simulink model "transformerlesspv0002"  (Simulink 9.2)
settings: Solver=ode45  StartTime=0.0  StopTime=2  RelTol=1e-3  EnableMultiTasking=on
undefined symbols (not defined in the file): dEgdT, EgRef, gcbh, k1, Rsh_array5pc, sps_rtmsupport, Tref_K, Ts_Control, VT_ref
libraries: powerlib x40, spsPVarrayModel x3, simulink x1, simulink_extras x1
(part 6 of 6)

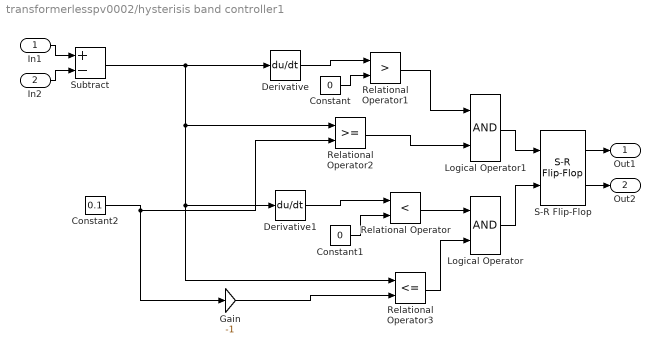
== system transformerlesspv0002/hysterisis band controller1 ==
  In1 : Inport
  In2 : Inport  Port=2
  Constant : Constant  Value=0
  Constant1 : Constant  Value=0
  Constant2 : Constant  Value=0.1
  Derivative : Derivative
  Derivative1 : Derivative
  Gain : Gain  Gain=-1
  Logical Operator : Logic  AllPortsSameDT=off  OutDataTypeStr=boolean
  Logical Operator1 : Logic  AllPortsSameDT=off  OutDataTypeStr=boolean
  Relational Operator : RelationalOperator  Operator=<  OutDataTypeStr=boolean  RndMeth=Nearest
  Relational Operator1 : RelationalOperator  Operator=>  OutDataTypeStr=boolean  RndMeth=Nearest
  Relational Operator2 : RelationalOperator  OutDataTypeStr=boolean  RndMeth=Nearest
  Relational Operator3 : RelationalOperator  Operator=<=  OutDataTypeStr=boolean  RndMeth=Nearest
  S-R Flip-Flop : simulink_extras/Flip Flops/S-R Flip-Flop  initial_condition=1
  Subtract : Sum  Inputs=+-
  Out1 : Outport
  Out2 : Outport  Port=2
  wires:
  Derivative/1 -> Relational Operator1/1
  Constant/1 -> Relational Operator1/2
  Derivative1/1 -> Relational Operator/1
  Constant1/1 -> Relational Operator/2
  Subtract/1 -> Derivative1/1, Relational Operator3/1, Relational Operator2/1, Derivative/1
  Relational Operator1/1 -> Logical Operator1/1
  Relational Operator2/1 -> Logical Operator1/2
  Relational Operator/1 -> Logical Operator/1
  Relational Operator3/1 -> Logical Operator/2
  Gain/1 -> Relational Operator3/2
  Constant2/1 -> Relational Operator2/2, Gain/1
  Logical Operator1/1 -> S-R Flip-Flop/1
  Logical Operator/1 -> S-R Flip-Flop/2
  In1/1 -> Subtract/1
  S-R Flip-Flop/1 -> Out1/1
  In2/1 -> Subtract/2
  S-R Flip-Flop/2 -> Out2/1

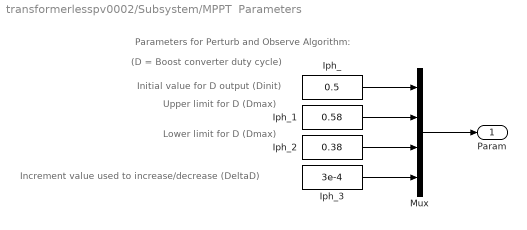
== system transformerlesspv0002/Subsystem/MPPT  Parameters ==
  note: Upper limit for D (Dmax)
  note: Increment value used to increase/decrease (DeltaD)
  note: Initial value for D output (Dinit)
  note: (D = Boost converter duty cycle)
  note: Lower limit for D (Dmax)
  note: Parameters for Perturb and Observe Algorithm:
  Iph_ : Constant  Value=0.5
  Iph_1 : Constant  Value=0.58
  Iph_2 : Constant  Value=0.38
  Iph_3 : Constant  Value=3e-4
  Mux : Mux
  Param : Outport
  wires:
  Iph_/1 -> Mux/1
  Iph_1/1 -> Mux/2
  Iph_2/1 -> Mux/3
  Iph_3/1 -> Mux/4
  Mux/1 -> Param/1

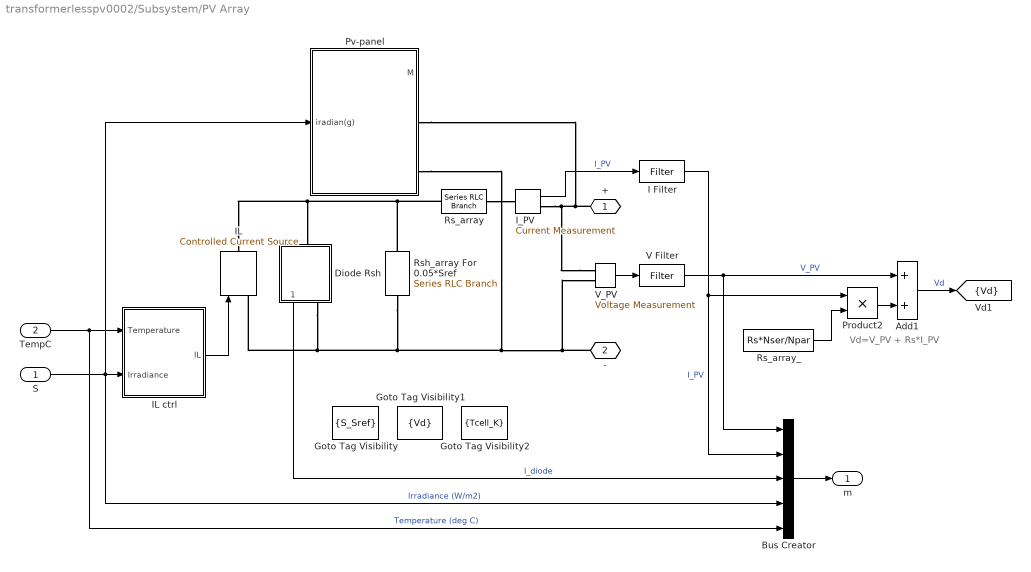
== system transformerlesspv0002/Subsystem/PV Array ==
  note: Vd=V_PV + Rs*I_PV
  S : Inport
  TempC : Inport  Port=2
  Add1 : Sum
  Bus Creator : BusCreator  Inputs=5
  Diode Rsh : Subsystem
      mask Display:
      | plot(-75,-50,100,150, [-15 -15 43 -15 -15 -75],[50 8 50 92 50 50], ...
      |     [43 43],[8 94],[100 43], [50 50])
  Goto Tag Visibility : GotoTagVisibility  GotoTag=S_Sref
  Goto Tag Visibility1 : GotoTagVisibility  GotoTag=Vd
  Goto Tag Visibility2 : GotoTagVisibility  GotoTag=Tcell_K
  I Filter : spsPVarrayModel/Filter  SystemSampleTime=-1  VariantControl=Variant1
  IL : powerlib/Electrical Sources/Controlled Current Source  Initialize=on  Source_Type=AC  Amplitude=0  Phase=0  Frequency=0  Measurements=None
      settings: SourceProductName=Simscape Electrical
  IL ctrl : Subsystem
  I_PV : powerlib/Measurements/Current Measurement  PhasorSimulation=off  OutputType=Complex  PSBequivalent=0
      settings: SourceProductName=Simscape Electrical
  Product2 : Product  Inputs=**  RndMeth=Zero
  Pv-panel : Subsystem  mask(PV_PANEL){Ns=600, Np=66}
      mask prompts: Ns "Number_of_series_connectd_pvcells"; Np "Number_of_parallel_connected_strings"
      mask help: THIS BLOCK IMPLEMENTS PHOTO VOLTAIC PANEL.NUMBER OF SERIES PV CELLS CAN BE CONTROLLED AND NUMBER OF PARALLEL STRINGS 0F PV CELLS CAN BE CONTROLLED
      mask init:
      | u=1.5;%diode 
      | k=1.3806e-23;%boltzman constant
      | T=298;%room temp
      | q=1.6022e-19;%charge
      | vt=(u*k*T)/q;
      | Vt_panel=vt*Ns;
      | Iph=8;
      | Iph_panel=Iph*Np;
      | I0=9.845e-7;
      | I0_panel=I0*Np;
      | Rs=0.001;
      | Rs_panel=Rs*(Ns/Np);
      | Rsh=142.94;
      | Rsh_panel=Rsh*(Ns/Np);
      | G0=1000;
      mask Display: image(imread('pv_panel.jpg'))
  Rs_array : powerlib/Elements/Series RLC Branch  LConnTagsString=__new0  RConnTagsString=__new0  BranchType=R  Resistance=Rs*Nser/Npar  Inductance=1e-3  SetiL0=off  InitialCurrent=0  Capacitance=1e-6  Setx0=off  InitialVoltage=0  Measurements=None
      settings: SourceProductName=Simscape Electrical
  Rs_array_ : Constant  Value=Rs*Nser/Npar
  Rsh_array For 0.05*Sref : powerlib/Elements/Series RLC Branch  LConnTagsString=__new0  RConnTagsString=__new0  BranchType=R  Resistance=Rsh_array5pc  Inductance=1e-3  SetiL0=off  InitialCurrent=0  Capacitance=1e-6  Setx0=off  InitialVoltage=0  Measurements=None
      settings: SourceProductName=Simscape Electrical
  V Filter : spsPVarrayModel/Filter  SystemSampleTime=-1  VariantControl=Variant1
  V_PV : powerlib/Measurements/Voltage Measurement  PhasorSimulation=off  OutputType=Complex  PSBequivalent=0
      settings: SourceProductName=Simscape Electrical
  + : PMIOPort  Side=Right
  - : PMIOPort  Port=2  Side=Right
  m : Outport
  tag scope: Vd=scoped
  wires:
  V Filter/1 -> Add1/1, Bus Creator/1  "V_PV"
  I Filter/1 -> Product2/1, Bus Creator/2  "I_PV"
  V_PV/1 -> V Filter/1
  IL ctrl/1(IL) -> IL/1
  Bus Creator/1 -> m/1
  Rs_array_/1 -> Product2/2
  Product2/1 -> Add1/2
  I_PV/1 -> I Filter/1  "I_PV"
  Add1/1 -> [Vd]  "Vd"
  Diode Rsh/1(Idiode) -> Bus Creator/3  "I_diode"
  S/1 -> Bus Creator/4, Pv-panel/1(iradian(g)), IL ctrl/2(Irradiance)  "Irradiance (W/m2)"
  TempC/1 -> IL ctrl/1(Temperature), Bus Creator/5  "Temperature (deg C)"
  connections:
  Rs_array/RConn1 -- I_PV/LConn1
  IL/LConn1 -- Diode Rsh/RConn1 -- Rsh_array For 0.05*Sref/RConn1 -- -/RConn1 -- V_PV/LConn2 -- Pv-panel/RConn2
  IL/RConn1 -- Rsh_array For 0.05*Sref/LConn1 -- Rs_array/LConn1 -- Diode Rsh/LConn1
  V_PV/LConn1 -- Pv-panel/RConn1 -- +/RConn1 -- I_PV/RConn1

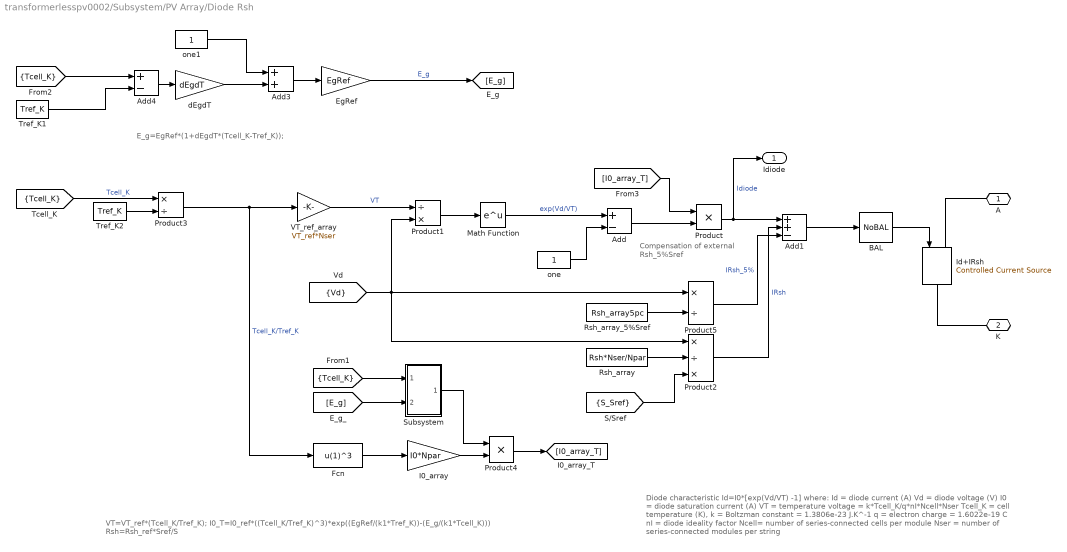
== system transformerlesspv0002/Subsystem/PV Array/Diode Rsh ==
  note: Compensation of
      | external Rsh_5%Sref
  note: Diode characteristic
      |    Id=I0*[exp(Vd/VT) -1]
      |
      | where:
      |      Id = diode current (A)
      |      Vd = diode voltage (V)
      |      I0 = diode saturation current (A)
      |      VT = temperature voltage = k*Tcell_K/q*nI*Ncell*Nser
      | Tcell_K = cell temperature (K),
      |       k = Boltzman constant = 1.3806e-23 J.K^-1
      |       q = electron charge = 1.6022e-19 C
      |      nI = diode ideality factor
      |    Ncell= number of series-connected cells per module
      |    Nser = number of series-connected modules per string
  note: VT=VT_ref*(Tcell_K/Tref_K);
      | I0_T=I0_ref*((Tcell_K/Tref_K)^3)*exp((EgRef/(k1*Tref_K))-(E_g/(k1*Tcell_K)))
      | Rsh=Rsh_ref*Sref/S
  note: E_g=EgRef*(1+dEgdT*(Tcell_K-Tref_K));
  Add : Sum  Inputs=+-
  Add1 : Sum  Inputs=++-
  Add3 : Sum
  Add4 : Sum  Inputs=+-
  BAL : spsPVarrayModel/NoBAL  SystemSampleTime=-1  VariantControl=NoBAL
  EgRef : Gain  Gain=EgRef
  Fcn : Fcn  Expr=u(1)^3
  I0_array : Gain  Gain=I0*Npar
  Id+IRsh : powerlib/Electrical Sources/Controlled Current Source  Initialize=on  Source_Type=AC  Amplitude=0  Phase=0  Frequency=0  Measurements=None
      settings: SourceProductName=Simscape Electrical
  Math Function : Math  SaturateOnIntegerOverflow=on
  Product : Product  RndMeth=Zero
  Product1 : Product  Inputs=/*  RndMeth=Zero
  Product2 : Product  Inputs=*/*  RndMeth=Zero
  Product3 : Product  Inputs=*/  RndMeth=Zero
  Product4 : Product  Inputs=**  RndMeth=Zero
  Product5 : Product  Inputs=*/  RndMeth=Zero
  Rsh_array : Constant  Value=Rsh*Nser/Npar
  Rsh_array_5%Sref : Constant  Value=Rsh_array5pc
  Subsystem : Subsystem
  Tref_K1 : Constant  Value=Tref_K
  Tref_K2 : Constant  Value=Tref_K
  VT_ref_array : Gain  Gain=VT_ref*Nser
  dEgdT : Gain  Gain=dEgdT
  one : Constant
  one1 : Constant
  A : PMIOPort  Side=Left
  K : PMIOPort  Port=2  Side=Right
  Idiode : Outport
  wires:
  BAL/1 -> Id+IRsh/1
  Add1/1 -> BAL/1
  Product5/1 -> Add1/3  "IRsh_5%"
  Rsh_array_5%Sref/1 -> Product5/2
  Math Function/1 -> Add/1  "exp(Vd/VT)"
  Product2/1 -> Add1/2  "IRsh"
  Product/1 -> Add1/1, Idiode/1  "Idiode"
  Product1/1 -> Math Function/1
  one/1 -> Add/2
  Rsh_array/1 -> Product2/2
  [Tcell_K] -> Product3/1  "Tcell_K"
  Product3/1 -> VT_ref_array/1, Fcn/1  "Tcell_K/Tref_K"
  one1/1 -> Add3/1
  Add4/1 -> dEgdT/1
  dEgdT/1 -> Add3/2
  Add3/1 -> EgRef/1
  EgRef/1 -> [E_g]  "E_g"
  I0_array/1 -> Product4/2
  Fcn/1 -> I0_array/1
  [Tcell_K] -> Add4/1
  Tref_K1/1 -> Add4/2
  Subsystem/1(exp) -> Product4/1
  [Tcell_K] -> Subsystem/1(Tcell_K)
  [E_g] -> Subsystem/2(E_g)
  Tref_K2/1 -> Product3/2
  Product4/1 -> [I0_array_T]
  Add/1 -> Product/2
  VT_ref_array/1 -> Product1/1  "VT"
  [I0_array_T] -> Product/1
  [S_Sref] -> Product2/3
  [Vd] -> Product5/1, Product2/1, Product1/2
  connections:
  Id+IRsh/RConn1 -- K/RConn1
  A/RConn1 -- Id+IRsh/LConn1

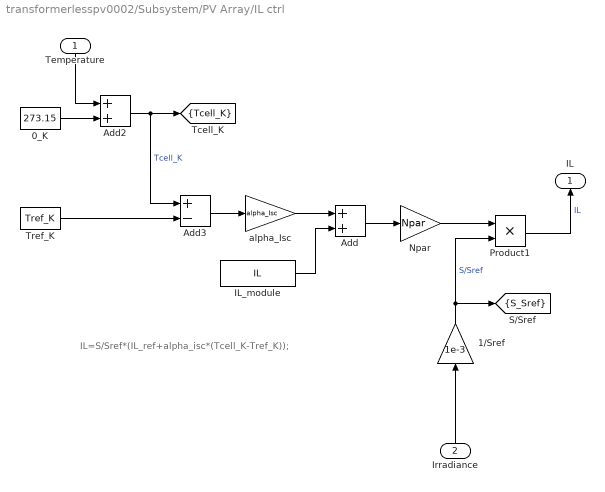
== system transformerlesspv0002/Subsystem/PV Array/IL ctrl ==
  note: IL=S/Sref*(IL_ref+alpha_isc*(Tcell_K-Tref_K));
  Temperature : Inport
  Irradiance : Inport  Port=2
  0_K : Constant  Value=273.15
  1/Sref : Gain  Gain=1e-3
  Add : Sum
  Add2 : Sum
  Add3 : Sum  Inputs=+-
  IL_module : Constant  Value=IL
  Npar : Gain  Gain=Npar
  Product1 : Product  Inputs=**  RndMeth=Zero
  Tref_K : Constant  Value=Tref_K
  alpha_Isc : Gain  Gain=alpha_Isc
  IL : Outport
  tag scope: S_Sref=scoped, Tcell_K=scoped
  wires:
  Temperature/1 -> Add2/1
  Irradiance/1 -> 1/Sref/1
  alpha_Isc/1 -> Add/1
  Add3/1 -> alpha_Isc/1
  Tref_K/1 -> Add3/2
  Product1/1 -> IL/1  "IL"
  IL_module/1 -> Add/2
  0_K/1 -> Add2/2
  Add/1 -> Npar/1
  Add2/1 -> Add3/1, [Tcell_K]  "Tcell_K"
  Npar/1 -> Product1/1
  1/Sref/1 -> Product1/2, [S_Sref]  "S/Sref"

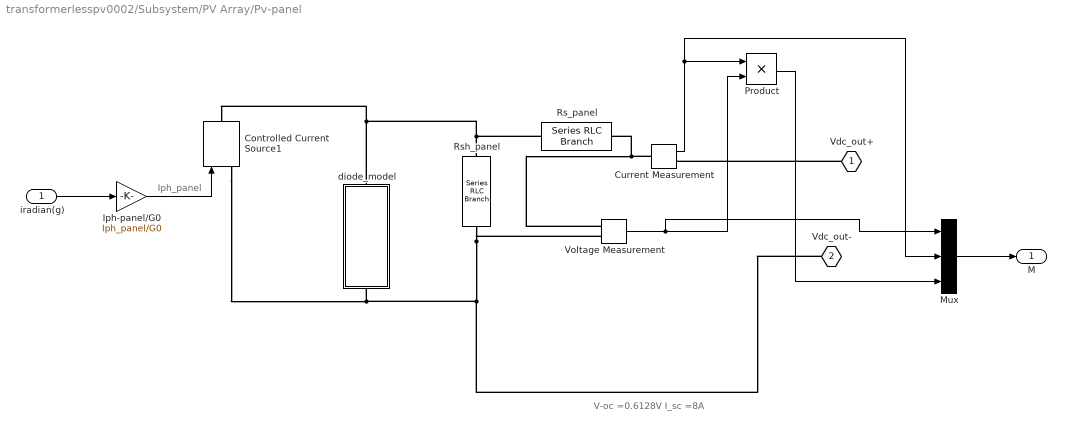
== system transformerlesspv0002/Subsystem/PV Array/Pv-panel ==
  note: V-oc =0.6128V
      | I_sc =8A
  note: Iph_panel
  iradian(g) : Inport
  Controlled Current Source1 : powerlib/Electrical Sources/Controlled Current Source  Initialize=on  Source_Type=AC  Amplitude=0  Phase=0  Frequency=0  Measurements=None
      settings: SourceProductName=Simscape Electrical
  Current Measurement : powerlib/Measurements/Current Measurement  PhasorSimulation=off  OutputType=Complex  PSBequivalent=0
      settings: SourceProductName=Simscape Electrical
  Iph-panel/G0 : Gain  Gain=Iph_panel/G0
  Mux : Mux  Inputs=3
  Product : Product
  Rs_panel : powerlib/Elements/Series RLC Branch  LConnTagsString=__new0  RConnTagsString=__new0  BranchType=R  Resistance=Rs_panel  Inductance=1e-3  SetiL0=off  InitialCurrent=0  Capacitance=1e-6  Setx0=off  InitialVoltage=0  Measurements=None
      settings: SourceProductName=Simscape Electrical
  Rsh_panel : powerlib/Elements/Series RLC Branch  LConnTagsString=__new0  RConnTagsString=__new0  BranchType=R  Resistance=Rsh_panel  Inductance=1e-3  SetiL0=off  InitialCurrent=0  Capacitance=1e-6  Setx0=off  InitialVoltage=0  Measurements=None
      settings: SourceProductName=Simscape Electrical
  Voltage Measurement : powerlib/Measurements/Voltage Measurement  PhasorSimulation=off  OutputType=Complex  PSBequivalent=0
      settings: SourceProductName=Simscape Electrical
  diode_model : Subsystem
      mask Display: plot([2,2,1,2,3,1,2,1,3,2,2],[4,3,3,2,3,3,2,2,2,2,1])
  Vdc_out+ : PMIOPort  Side=Right
  Vdc_out- : PMIOPort  Port=2  Side=Right
  M : Outport
  wires:
  iradian(g)/1 -> Iph-panel/G0/1
  Iph-panel/G0/1 -> Controlled Current Source1/1
  Current Measurement/1 -> Mux/2, Product/1
  Voltage Measurement/1 -> Mux/1, Product/2
  Product/1 -> Mux/3
  Mux/1 -> M/1
  connections:
  Vdc_out+/RConn1 -- Current Measurement/RConn1
  Controlled Current Source1/RConn1 -- diode_model/LConn1 -- Rsh_panel/LConn1 -- Rs_panel/RConn1
  Voltage Measurement/LConn1 -- Current Measurement/LConn1 -- Rs_panel/LConn1
  Controlled Current Source1/LConn1 -- diode_model/RConn1 -- Vdc_out-/RConn1 -- Voltage Measurement/LConn2 -- Rsh_panel/RConn1

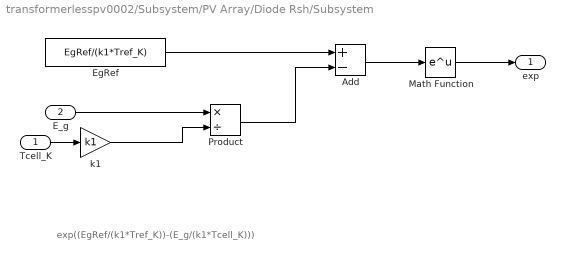
== system transformerlesspv0002/Subsystem/PV Array/Diode Rsh/Subsystem ==
  note: exp((EgRef/(k1*Tref_K))-(E_g/(k1*Tcell_K)))
  Tcell_K : Inport
  E_g : Inport  Port=2
  Add : Sum  Inputs=+-
  EgRef : Constant  Value=EgRef/(k1*Tref_K)
  Math Function : Math  SaturateOnIntegerOverflow=on
  Product : Product  Inputs=*/
  k1 : Gain  Gain=k1
  exp : Outport
  wires:
  EgRef/1 -> Add/1
  E_g/1 -> Product/1
  Tcell_K/1 -> k1/1
  k1/1 -> Product/2
  Product/1 -> Add/2
  Add/1 -> Math Function/1
  Math Function/1 -> exp/1

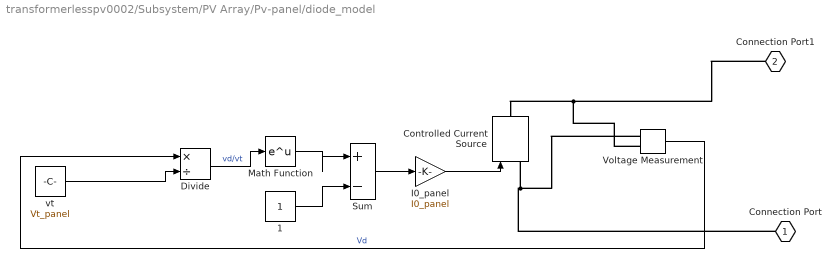
== system transformerlesspv0002/Subsystem/PV Array/Pv-panel/diode_model ==
  1 : Constant
  Controlled Current Source : powerlib/Electrical Sources/Controlled Current Source  Initialize=on  Source_Type=AC  Amplitude=0  Phase=0  Frequency=0  Measurements=None
      settings: SourceProductName=Simscape Electrical
  Divide : Product  Inputs=*/
  I0_panel : Gain  Gain=I0_panel
  Math Function : Math  SaturateOnIntegerOverflow=on
  Sum : Sum  Inputs=|+-
  Voltage Measurement : powerlib/Measurements/Voltage Measurement  PhasorSimulation=off  OutputType=Complex  PSBequivalent=0
      settings: SourceProductName=Simscape Electrical
  vt : Constant  Value=Vt_panel
  Connection Port : PMIOPort  Side=Left
  Connection Port1 : PMIOPort  Port=2  Side=Right
  wires:
  vt/1 -> Divide/2
  Divide/1 -> Math Function/1  "vd/vt"
  Math Function/1 -> Sum/1
  1/1 -> Sum/2
  Sum/1 -> I0_panel/1
  I0_panel/1 -> Controlled Current Source/1
  Voltage Measurement/1 -> Divide/1  "Vd"
  connections:
  Voltage Measurement/LConn2 -- Connection Port1/RConn1 -- Controlled Current Source/RConn1
  Voltage Measurement/LConn1 -- Connection Port/RConn1 -- Controlled Current Source/LConn1

== matlab function Subsystem/MPPT Control (Perturb & Observe MPPT)  ==
  settings: updateMethod=DISCRETE  sampleTime=Ts_Control
  data: Param input double; Enabled input double; V input double =V; I input double; D output double
function D  = PandO(Param, Enabled, V, I)

% MPPT controller based on the Perturb & Observe algorithm.

% D output = Duty cycle of the boost converter (value between 0 and 1)
%
% Enabled input = 1 to enable the MPPT controller
% V input = PV array terminal voltage (V)
% I input = PV array current (A)
%
% Param input:
Dinit = Param(1);  %Initial value for D output
Dmax = Param(2);   %Maximum value for D
Dmin = Param(3);   %Minimum value for D
deltaD = Param(4); %Increment value used to increase/decrease the duty cycle D
% ( increasing D = decreasing Vref )
%  

persistent Vold Pold Dold;

dataType = 'double';

if isempty(Vold)
    Vold=0;
    Pold=0;
    Dold=Dinit;
end
P= V*I;
dV= V - Vold;
dP= P - Pold;

if dP ~= 0 & Enabled ~=0
    if dP < 0
        if dV < 0
            D = Dold - deltaD;
        else
            D = Dold + deltaD;
        end
    else
        if dV < 0
            D = Dold + deltaD;
        else
            D = Dold - deltaD;
        end    
    end
else D=Dold;
end

if D >= Dmax | D<= Dmin
    D=Dold;
end

Dold=D;
Vold=V;
Pold=P;
